simulink model "trefas"  (R2020b)
settings: Solver=VariableStepAuto  StartTime=0.0  StopTime=stop_time  RelTol=tolerance
model workspace (MAT data in the model file):
  R = 40
  a = 220
  freq = 314.16
values from neighbouring files (symbols this model uses):
  amplitude = 220    [lab1.m]
  L = 95 * 10^-3    (= 0.095)    [lab1.m]
  phase_1 = 0    [lab1.m]
  phase_2 = 2*pi / 3    (= 2.09439510239)    [lab1.m]
  phase_3 = 4*pi / 3    (= 4.18879020479)    [lab1.m]
settings Model: Creator=axelfroborg  LastModifiedBy=axelfroborg

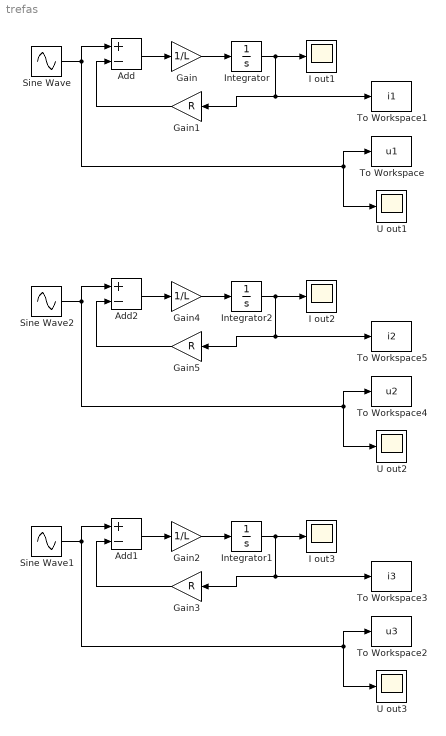
== system trefas ==
  Add : Sum  Inputs=+-
  Add1 : Sum  Inputs=+-
  Add2 : Sum  Inputs=+-
  Gain : Gain  Gain=1/L
  Gain1 : Gain  Gain=R
  Gain2 : Gain  Gain=1/L
  Gain3 : Gain  Gain=R
  Gain4 : Gain  Gain=1/L
  Gain5 : Gain  Gain=R
  I out1 : Scope
  I out2 : Scope
  I out3 : Scope
  Integrator : Integrator
  Integrator1 : Integrator
  Integrator2 : Integrator
  Sine Wave : Sin  Amplitude=amplitude  Frequency=freq  Phase=phase_1  SampleTime=0
  Sine Wave1 : Sin  Amplitude=amplitude  Frequency=freq  Phase=phase_3  SampleTime=0
  Sine Wave2 : Sin  Amplitude=amplitude  Frequency=freq  Phase=phase_2  SampleTime=0
  To Workspace : ToWorkspace  VariableName=u1  SampleTime=-1
  To Workspace1 : ToWorkspace  VariableName=i1  SampleTime=-1
  To Workspace2 : ToWorkspace  VariableName=u3  SampleTime=-1
  To Workspace3 : ToWorkspace  VariableName=i3  SampleTime=-1
  To Workspace4 : ToWorkspace  VariableName=u2  SampleTime=-1
  To Workspace5 : ToWorkspace  VariableName=i2  SampleTime=-1
  U out1 : Scope
  U out2 : Scope
  U out3 : Scope
  wires:
  Integrator/1 -> Gain1/1, To Workspace1/1, I out1/1
  Add/1 -> Gain/1
  Gain/1 -> Integrator/1
  Gain1/1 -> Add/2
  Sine Wave/1 -> U out1/1, To Workspace/1, Add/1
  Gain4/1 -> Integrator2/1
  Add2/1 -> Gain4/1
  Gain5/1 -> Add2/2
  Integrator2/1 -> Gain5/1, To Workspace5/1, I out2/1
  Sine Wave2/1 -> U out2/1, To Workspace4/1, Add2/1
  Gain2/1 -> Integrator1/1
  Add1/1 -> Gain2/1
  Gain3/1 -> Add1/2
  Integrator1/1 -> Gain3/1, To Workspace3/1, I out3/1
  Sine Wave1/1 -> U out3/1, To Workspace2/1, Add1/1
